simulink model "Load_Simulation_01"  (R2017a)
settings: Solver=VariableStepAuto  StartTime=0.0  StopTime=3600
undefined symbols (not defined in the file or in its folder): sigbuilder_block
settings Model: Creator=hlope  LastModifiedBy=hlope

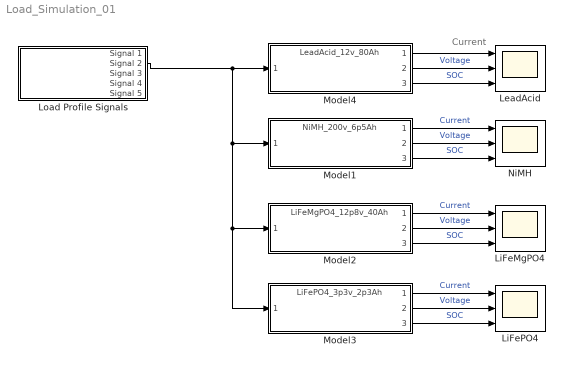
== system Load_Simulation_01 ==
  note: Current
  LeadAcid : Scope  NumInputPorts=3
  LiFeMgPO4 : Scope  NumInputPorts=3
  LiFePO4 : Scope  NumInputPorts=3
  Load Profile Signals : Subsystem  Tag=STV Subsys  LoadFcn=sigbuilder_block('load');  StartFcn=sigbuilder_block('start');  StopFcn=sigbuilder_block('stop');  ClipboardFcn=sigbuilder_block('clipboard');  mask(Sigbuilder block){tuvar=[0:10]}
      mask help: Simulink:masks:SigbuilderBlock_MD
      mask init:
      | if ~strcmp(get_param(bdroot(gcbh),'SimulationStatus'),'stopped') tuvar = sigbuilder_block('maskInit'); end
      settings: CopyFcn=sigbuilder_block('copy');  DeleteFcn=sigbuilder_block('delete');  ModelCloseFcn=sigbuilder_block('modelClose');  PreSaveFcn=sigbuilder_block('preSave');  PauseFcn=sigbuilder_block('pause');  ContinueFcn=sigbuilder_block('continue');  NameChangeFcn=sigbuilder_block('namechange');  OpenFcn=sigbuilder_block('open',[463.8 -22.2 574.8 516.6 ]);  CloseFcn=sigbuilder_block('close');
      mask Display: plot(0, 0, 100, 100,[2, 2, 32, 32, 2], [68, 8, 8, 68, 68],[32, 2], [38, 38], [32, 19, 2],[53, 60, 44], [32, 17, 17, 2],[16, 16, 31, 31]);txt = getActiveGroup(gcbh);text(2, 100, txt,'verticalAlignment', 'top');
  Model1 : ModelReference  ModelNameDialog=NiMH_200v_6p5Ah.slx  SimulationMode=Normal  ModelReferenceVersion=1.140
  Model2 : ModelReference  ModelNameDialog=LiFeMgPO4_12p8v_40Ah.slx  SimulationMode=Normal  ModelReferenceVersion=1.147
  Model3 : ModelReference  ModelNameDialog=LiFePO4_3p3v_2p3Ah.slx  SimulationMode=Normal  ModelReferenceVersion=1.144
  Model4 : ModelReference  ModelNameDialog=LeadAcid_12v_80Ah.slx  SimulationMode=Normal  ModelReferenceVersion=1.142
  NiMH : Scope  NumInputPorts=3
  wires:
  Load Profile Signals/2(Signal 2) -> Model4/1, Model3/1, Model2/1, Model1/1
  Model4/2 -> LeadAcid/2  "Voltage"
  Model4/1 -> LeadAcid/1
  Model4/3 -> LeadAcid/3  "SOC"
  Model1/1 -> NiMH/1  "Current"
  Model1/2 -> NiMH/2  "Voltage"
  Model1/3 -> NiMH/3  "SOC"
  Model2/1 -> LiFeMgPO4/1  "Current"
  Model2/2 -> LiFeMgPO4/2  "Voltage"
  Model2/3 -> LiFeMgPO4/3  "SOC"
  Model3/1 -> LiFePO4/1  "Current"
  Model3/2 -> LiFePO4/2  "Voltage"
  Model3/3 -> LiFePO4/3  "SOC"

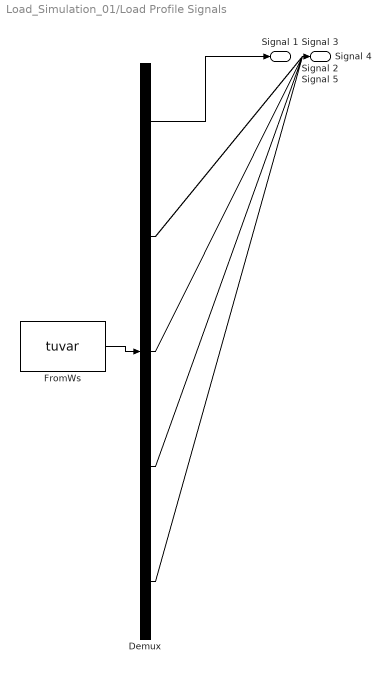
== system Load_Simulation_01/Load Profile Signals ==
  Demux : Demux  Tag=STV Demux  Outputs=5
  FromWs : FromWorkspace  Tag=STV FromWs  VariableName=tuvar  SampleTime=0
      SigBuilderData=|
      | common.afterFinalStr = 'Extrapolate'
      | common.sampleTime = 0
      | dataSet.timeRange = [0 3600]
      | dataSet.name = 'Group 1'
      | sbobj.Groups.Name = 'Group 1'
      | sbobj.Groups.Signals(1).Name = 'Signal 1'
      | sbobj.Groups.Signals(1).XData = [0 2000 2000 3000 3000 3600]
      | sbobj.Groups.Signals(1).YData = [1 1 0 0 1 1]
      | sbobj.Groups.Signals(2).Name = 'Signal 2'
      | sbobj.Groups.Signals(2).XData = [0 200 200 300 300 500 500 900 900 1000 1000 1100 1100 1500 1500 1900 1900 2200 2200 2500 2500 2600 2600 2700 2700 2800 2800 3000 3000 3100 3100 3500 3500 3600 3600]
      | sbobj.Groups.Signals(2).YData = [0 0 1 1 0 0 1 1 0 0 1 1 0 0 1 1 0 0 1 1 0 0 1 1 0 0 1 1 0 0 1 1 0 0 1]
      | sbobj.Groups.Signals(3).Name = 'Signal 3'
      | sbobj.Groups.Signals(3).XData = [0 0.5 0.5 1 1 1.5 1.5 2 2 2.5 2.5 3 3 3.5 3.5 4 4 4.5 4.5 5 5 5.5 5.5 6 6 6.5 6.5 7 7 7.5 7.5 8 8 8.5 8.5 9 9 9.5 9.5 3600]
      | sbobj.Groups.Signals(3).YData = [2 2 0 0 2 2 0 0 2 2 0 0 2 2 0 0 2 2 0 0 2 2 0 0 2 2 0 0 2 2 0 0 2 2 0 0 2 2 0 0]
      | sbobj.Groups.Signals(4).Name = 'Signal 4'
      | sbobj.Groups.Signals(4).XData = [0 3600]
      | sbobj.Groups.Signals(4).YData = [0 0]
      | sbobj.Groups.Signals(5).Name = 'Signal 5'
      | sbobj.Groups.Signals(5).XData = [0 100 100 200 200 300 300 400 400 500 500 700 700 900 900 1200 1200 1300 1300 1400 1400 1500 1500 2000 2000 2200 2200 2300 2300 2800 2800 2900 2900 3000 3000 3300 3300 3400 3400 3500 3500 3600]
      | sbobj.Groups.Signals(5).YData = [1 1 0 0 1 1 0 0 1 1 0 0 1 1 0 0 1 1 0 0 1 1 0 0 1 1 0 0 1 1 0 0 1 1 0 0 1 1 0 0 1 1]
      | sbobj.Groups.TimeRange = [0 3600]
  Signal 1 : Outport  Tag=STV Outport
  Signal 2 : Outport  Tag=STV Outport  Port=2
  Signal 3 : Outport  Tag=STV Outport  Port=3
  Signal 4 : Outport  Tag=STV Outport  Port=4
  Signal 5 : Outport  Tag=STV Outport  Port=5
  wires:
  Demux/1 -> Signal 1/1
  FromWs/1 -> Demux/1
  Demux/2 -> Signal 2/1
  Demux/3 -> Signal 3/1
  Demux/4 -> Signal 4/1
  Demux/5 -> Signal 5/1
